simulink model "ASML_Simulate"  (R2022a)
settings: Solver=FixedStepAuto  StartTime=0.0  StopTime=1  FixedStep=Ts  RelTol=1e-3
model workspace (MAT data in the model file):
  enab = 1
  eol = 6
  euvTarget = Simulink.Parameter
  euvTarget.Value = 4.4
  euvTarget.DataType = 'auto'
  euvTarget.Complexity = 'real'
  euvTarget.Dimensions = [1 1]
values from neighbouring files (symbols this model uses):
  euvTarget = 5    [modelParams.mat]
  HitDelayMode = 'zeroShot'    [modelParams.mat]    (also in variantParams.mat)
  SenseDelayMode = 'twoShot'    [modelParams.mat]    (also in variantParams.mat)
  Ts = 20e-6    (= 2e-05)    [computeDose1Burst.m]    (also in computeDose1Burst_filtered.m; modelParams.mat)
libraries: simulink x1
settings Model: Creator=rjacques  LastModifiedBy=maxcr
settings SolverCC: AlgebraicLoopSolver=TrustRegion
settings DataIOCC: ExternalInput=extInput_SimulateEuvControl  DSMLogging=off  SaveTime=off  ReturnWorkspaceOutputs=off
settings OptimizationCC: EfficientMapNaN2IntZero=off
settings DebuggingCC: AlgebraicLoopMsg=none  UnconnectedInputMsg=warning  UnconnectedOutputMsg=warning  UnconnectedLineMsg=warning  SFMachineParentedDataDiag=warning  ArithmeticOperatorsInVariantConditions=warning
settings HardwareCC: TargetBitPerPointer=64  TargetBitPerSizeT=64  TargetBitPerPtrDiffT=64  TargetLongLongMode=on  TargetIntDivRoundTo=Zero  TargetEndianess=LittleEndian  TargetWordSize=64  TargetHWDeviceType=MATLAB Host  ProdEqTarget=off
settings SFSimCC: SimUseLocalCustomCode=off  CustomCodeUndefinedFunction=UseInterfaceOnly
settings RTWCC: SystemTargetFile=accel.tlc  TemplateMakefile=accel_default_tmf  RTWVerbose=off  DLArmComputeVersion=19.05
settings CodeAppCC: MaxIdLength=128
settings STFCustomTargetCC: ConcurrentExecutionCompliant=on  MATLABClassNameForMDSCustomization=Simulink.SoftwareTarget.TargetSpecificTriggerConfigurationBase  SystemTargetFile=accel.tlc

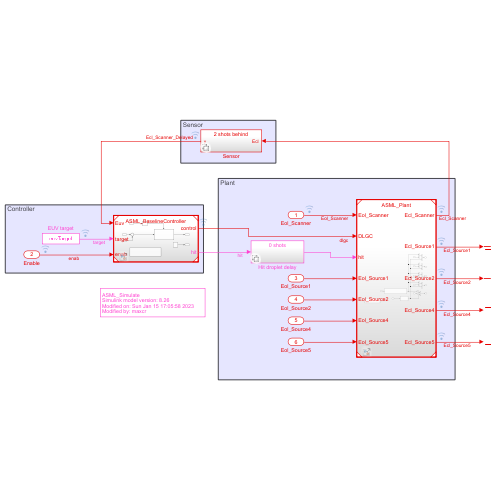
[thumbnail: Simulink's stored preview of the top-level diagram]
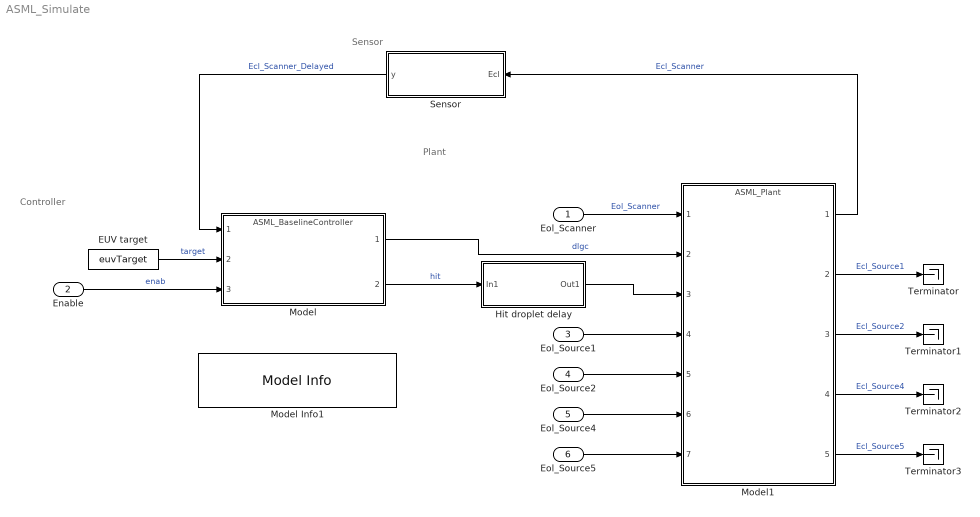
== system ASML_Simulate ==
  note: Sensor
  note: Controller
  note: Plant
  Eol_Scanner : Inport  OutDataTypeStr=double  SampleTime=Ts
  Enable : Inport  Port=2  OutDataTypeStr=double  SampleTime=Ts
  Eol_Source1 : Inport  Port=3  OutDataTypeStr=double  SampleTime=Ts
  Eol_Source2 : Inport  Port=4  OutDataTypeStr=double  SampleTime=Ts
  Eol_Source4 : Inport  Port=5  OutDataTypeStr=double  SampleTime=Ts
  Eol_Source5 : Inport  Port=6  OutDataTypeStr=double  SampleTime=Ts
  EUV target : Constant  Value=euvTarget  OutDataTypeStr=double
  Hit droplet delay : Subsystem  Variant=on
  Model : ModelReference  ModelNameDialog=ASML_BaselineController.slx  SimulationMode=Normal  ModelReferenceVersion=5.24
  Model Info1 : simulink/Model-Wide Utilities/Model Info  Frame=on  DisplayStringWithTags=|  HorizontalTextAlignment=Left  LeftAlignmentValue=0.02
      | %<ModelName>
      | Simulink model version: %<ModelVersion>
      | Modified on: %<LastModificationDate>
      | Modified by: %<ModifiedBy>
  Model1 : ModelReference  ModelNameDialog=ASML_Plant.slx  SimulationMode=Normal  ModelReferenceVersion=8.20
  Sensor : Subsystem  Variant=on  VariantControl=Variant1
  Terminator{,1..3} (4 alike) : Terminator
  wires:
  Model/1 -> Model1/2  "dlgc"
  Eol_Scanner/1 -> Model1/1  "Eol_Scanner"
  EUV target/1 -> Model/2  "target"
  Model1/1 -> Sensor/1("Ecl ")  "Ecl_Scanner"
  Model/2 -> Hit droplet delay/1(In1)  "hit"
  Hit droplet delay/1(Out1) -> Model1/3
  Sensor/1(" y") -> Model/1  "Ecl_Scanner_Delayed"
  Enable/1 -> Model/3  "enab"
  Eol_Source1/1 -> Model1/4
  Eol_Source2/1 -> Model1/5
  Eol_Source4/1 -> Model1/6
  Eol_Source5/1 -> Model1/7
  Model1/3 -> Terminator1/1  "Ecl_Source2"
  Model1/4 -> Terminator2/1  "Ecl_Source4"
  Model1/5 -> Terminator3/1  "Ecl_Source5"
  Model1/2 -> Terminator/1  "Ecl_Source1"

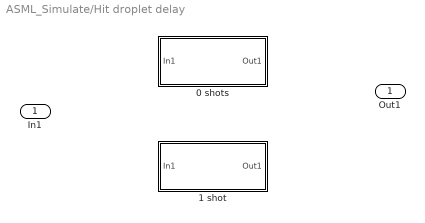
== system ASML_Simulate/Hit droplet delay ==
  In1 : Inport
  0 shots : Subsystem  VariantControl=strcmp(HitDelayMode,'zeroShot')
  1 shot : Subsystem  VariantControl=strcmp(HitDelayMode,'oneShot')
  Out1 : Outport  VectorParamsAs1DForOutWhenUnconnected=off

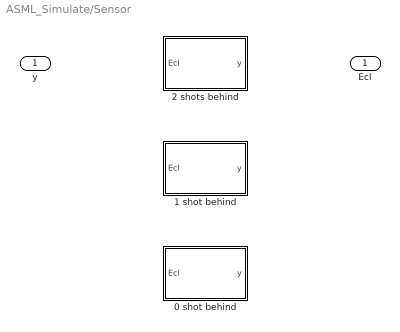
== system ASML_Simulate/Sensor ==
  "Ecl " : Inport
  0 shot behind : Subsystem  VariantControl=strcmp(SenseDelayMode,'zeroShot')
  1 shot behind : Subsystem  VariantControl=strcmp(SenseDelayMode,'oneShot')
  2 shots behind : Subsystem  VariantControl=strcmp(SenseDelayMode,'twoShot')
  " y" : Outport  VectorParamsAs1DForOutWhenUnconnected=off

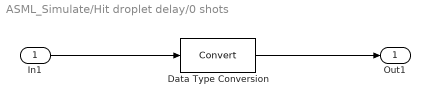
== system ASML_Simulate/Hit droplet delay/0 shots ==
  In1 : Inport
  Data Type Conversion : DataTypeConversion  SaturateOnIntegerOverflow=off  RndMeth=Floor
  Out1 : Outport  VectorParamsAs1DForOutWhenUnconnected=off
  wires:
  In1/1 -> Data Type Conversion/1
  Data Type Conversion/1 -> Out1/1

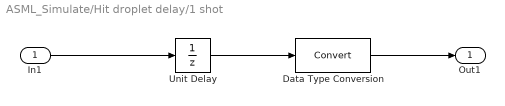
== system ASML_Simulate/Hit droplet delay/1 shot ==
  In1 : Inport
  Data Type Conversion : DataTypeConversion  SaturateOnIntegerOverflow=off  RndMeth=Floor
  Unit Delay : UnitDelay  InitialCondition=1  SampleTime=-1  HasFrameUpgradeWarning=on
  Out1 : Outport  VectorParamsAs1DForOutWhenUnconnected=off
  wires:
  Unit Delay/1 -> Data Type Conversion/1
  In1/1 -> Unit Delay/1
  Data Type Conversion/1 -> Out1/1

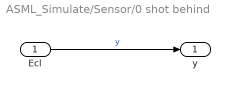
== system ASML_Simulate/Sensor/0 shot behind ==
  Ecl : Inport
  y : Outport  VectorParamsAs1DForOutWhenUnconnected=off
  wires:
  Ecl/1 -> y/1  "y"

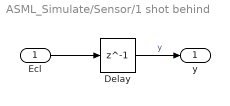
== system ASML_Simulate/Sensor/1 shot behind ==
  Ecl : Inport
  Delay : Delay  DelayLength=1  InitialCondition=5
  y : Outport  VectorParamsAs1DForOutWhenUnconnected=off
  wires:
  Ecl/1 -> Delay/1
  Delay/1 -> y/1  "y"

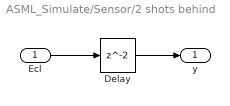
== system ASML_Simulate/Sensor/2 shots behind ==
  Ecl : Inport
  Delay : Delay  InitialCondition=5
  y : Outport  VectorParamsAs1DForOutWhenUnconnected=off
  wires:
  Delay/1 -> y/1
  Ecl/1 -> Delay/1
